simulink model "trafo1"  (Simulink 6.5)
settings: Solver=ode23t  StartTime=0.0  StopTime=1  RelTol=1e-3
undefined symbols (not defined in the file): powergui
libraries: powerlib x12, powerlib_extras x6
settings Model: Creator=RS  LastModifiedBy=RS

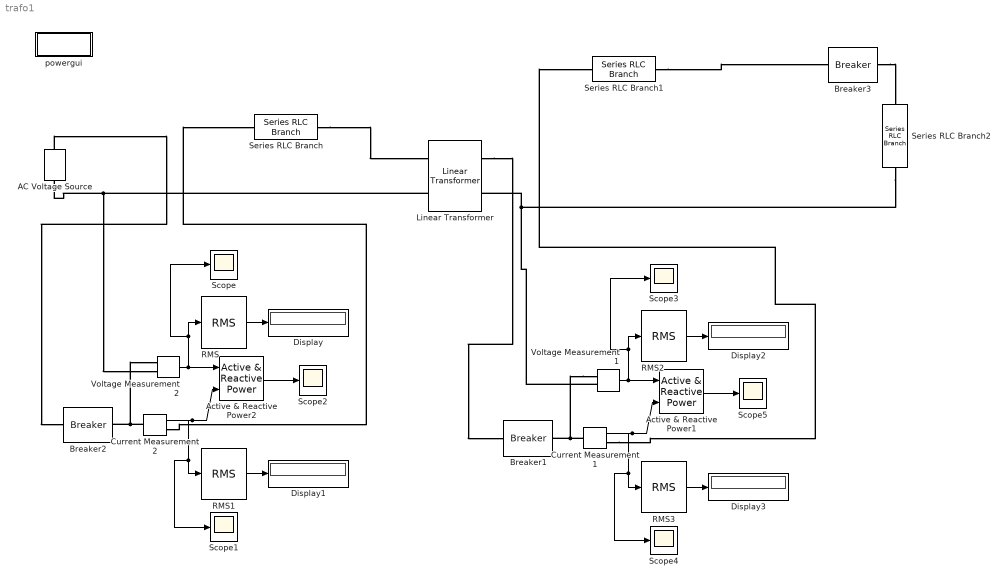
== system trafo1 ==
  AC Voltage Source : powerlib/Electrical Sources/AC Voltage Source  Orientation=up  DialogController=PMDialogs.PMDefaultMaskDlg  SystemSampleTime=-1  Amplitude=18172  Phase=0  Frequency=60  SampleTime=0  Measurements=None
  Active & Reactive Power1 : powerlib_extras/Measurements/Active & Reactive Power  DialogController=PMDialogs.PMDefaultMaskDlg  SystemSampleTime=-1  f1=60
  Active & Reactive Power2 : powerlib_extras/Measurements/Active & Reactive Power  DialogController=PMDialogs.PMDefaultMaskDlg  SystemSampleTime=-1  f1=60
  Breaker1 : powerlib/Elements/Breaker  DialogController=PMDialogs.PMDefaultMaskDlg  SystemSampleTime=-1  BreakerResistance=0.0001  InitialState=0  SnubberResistance=1e6  SnubberCapacitance=inf  SwitchingTimes="[ 0   2 ]"  External=off  Measurements=None  MoreParameters=off  NoBreakLoop=off
  Breaker2 : powerlib/Elements/Breaker  DialogController=PMDialogs.PMDefaultMaskDlg  SystemSampleTime=-1  BreakerResistance=0.0001  InitialState=0  SnubberResistance=1e6  SnubberCapacitance=inf  SwitchingTimes="[ 0   2 ]"  External=off  Measurements=None  MoreParameters=off  NoBreakLoop=off
  Breaker3 : powerlib/Elements/Breaker  DialogController=PMDialogs.PMDefaultMaskDlg  SystemSampleTime=-1  BreakerResistance=0.0001  InitialState=0  SnubberResistance=1e6  SnubberCapacitance=inf  SwitchingTimes="[ 0   2 ]"  External=off  Measurements=None  MoreParameters=off  NoBreakLoop=off
  Current Measurement1 : powerlib/Measurements/Current Measurement  DialogController=PMDialogs.PMDefaultMaskDlg  SystemSampleTime=-1  PhasorSimulation=off  OutputType=Complex  PSBequivalent=0
  Current Measurement2 : powerlib/Measurements/Current Measurement  DialogController=PMDialogs.PMDefaultMaskDlg  SystemSampleTime=-1  PhasorSimulation=off  OutputType=Complex  PSBequivalent=0
  Display{,1..3} (4 alike) : Display
  Linear Transformer : powerlib/Elements/Linear Transformer  DialogController=PMDialogs.PMDefaultMaskDlg  PhysicalDomain=powersysdomain  SubClassName=unknown  LeftPortType=p1  RightPortType=p1  LConnTagsString=a|b  RConnTagsString=A|B  UNITS=SI  NominalPower=[ 100000 60 ]  winding1="[12000    7.55      0.095875]"  winding2="[2400   0.302     0.003835]"  ThreeWindings=off  winding3=[3.15e+005 0.7938 0.084225]  RmLm="[99999999   99999999]"  Measurements=None  DataType=on
  RMS{,1..3} (4 alike) : powerlib_extras/Measurements/RMS  DialogController=PMDialogs.PMDefaultMaskDlg  SystemSampleTime=-1  f1=60
  Scope{,1..5} (6 alike) : Scope
      Scope settings: MaxDataPoints=10000000  SampleInput=on  SampleTime=10e-6
      Scope1 settings: MaxDataPoints=10000000  SampleInput=on  SampleTime=10e-6
      Scope2 settings: SaveName=ScopeData2  MaxDataPoints=10000000  SampleInput=on  SampleTime=10e-6
      Scope3 settings: SaveName=ScopeData3  MaxDataPoints=10000000  SampleInput=on  SampleTime=10e-6
      Scope4 settings: SaveName=ScopeData4  MaxDataPoints=10000000  SampleInput=on  SampleTime=10e-6
      Scope5 settings: SaveName=ScopeData5  MaxDataPoints=10000000  SampleInput=on  SampleTime=10e-6
  Series RLC Branch : powerlib/Elements/Series RLC Branch  DialogController=PMDialogs.PMDefaultMaskDlg  PhysicalDomain=powersysdomain  SubClassName=unknown  LeftPortType=p1  RightPortType=p1  LConnTagsString=__new0  RConnTagsString=__new0  BranchType=RL  Resistance=15.1  Inductance=0.17  SetiL0=off  InitialCurrent=0  Capacitance=1e-6  Setx0=off  InitialVoltage=0  Measurements=None
  Series RLC Branch1 : powerlib/Elements/Series RLC Branch  DialogController=PMDialogs.PMDefaultMaskDlg  PhysicalDomain=powersysdomain  SubClassName=unknown  LeftPortType=p1  RightPortType=p1  LConnTagsString=__new0  RConnTagsString=__new0  BranchType=RL  Resistance=1.27  Inductance=0.0047  SetiL0=off  InitialCurrent=0  Capacitance=1e-6  Setx0=off  InitialVoltage=0  Measurements=None
  Series RLC Branch2 : powerlib/Elements/Series RLC Branch  Orientation=down  DialogController=PMDialogs.PMDefaultMaskDlg  PhysicalDomain=powersysdomain  SubClassName=unknown  LeftPortType=p1  RightPortType=p1  LConnTagsString=__new0  RConnTagsString=__new0  BranchType=RL  Resistance=44.045  Inductance=0.0877  SetiL0=off  InitialCurrent=0  Capacitance=1e-6  Setx0=off  InitialVoltage=0  Measurements=None
  Voltage Measurement1 : powerlib/Measurements/Voltage Measurement  DialogController=PMDialogs.PMDefaultMaskDlg  SystemSampleTime=-1  PhasorSimulation=off  OutputType=Complex  PSBequivalent=0
  Voltage Measurement2 : powerlib/Measurements/Voltage Measurement  DialogController=PMDialogs.PMDefaultMaskDlg  SystemSampleTime=-1  PhasorSimulation=off  OutputType=Complex  PSBequivalent=0
  powergui : Subsystem  AncestorBlock=powerlib/powergui  InitFcn=powergui( 'InitFcn_Callback' , gcb , 0 , [ ] );  mask(PSB option menu block){SimulationMode=Continuous, SampleTime=50e-6, echomessages=off, RestoreLinks=warning, x0status=blocks, Frange=[0:2:500], Ylog=off, Xlog=on, ShowGrid=off, save=off, variable=ZData, structure=, ZoomFFT=on, StartTime=0.0, cycles=1, DisplayStyle=1, fundamental=60, FreqAxis=off, MaxFrequency=1000, frequencyindice=60, frequencyindicesteady=1, RmsSteady=1, display=off, Ts=0, frequency=60, methode=off, HookPort=off, Interpol=off}
      mask prompts: SimulationMode "Simulation mode"; SampleTime "Sample time Ts (when simulation mode is Discrete) (s)"; echomessages "Echo  Messages"; RestoreLinks "Restore disabled links"; x0status "Initial electrical states status"; Frange "Impedance tool: Frequency Range"; Ylog "Impedance tool: Log impedance"; Xlog "Impedance tool: log Frequency"; ShowGrid "Impedance tool: grid"; save "Impedance tool: Save Data To Workspace"; variable "Impedance tool: Variable Name"; structure "Structure Name (PSBFFTSCOPE)"; ZoomFFT "ZoomFFT (PSBFFTSCOPE)"; StartTime "Start Time (PSBFFTSCOPE)"; cycles "Cycles (PSBFFTSCOPE)"; DisplayStyle "Display style (PSBFFTSCOPE)"; fundamental "Fundamental (PSBFFTSCOPE)"; FreqAxis "Frequency Axis (PSBFFTSCOPE)"; MaxFrequency "Max Frequency (PSBFFTSCOPE)"; frequencyindice "Load flow frequency (Hz)"; frequencyindicesteady "Frequency indice (STEADYSTATE)"; RmsSteady "RMS display (STEADYSTATE)"; display "Display Results"; Ts "OBSOLETE 1"; frequency "Phasor frequency (Hz)"; methode "Phasor simulation"; HookPort "Hook port"; Interpol "Interpolate"
      mask init:
      | powerlibroot = which('powersysdomain');
      | PSBroot = powerlibroot(1:end-16);
      | %
      | switch SimulationMode
      | 	case 1
      | 		message=sprintf('Continuous');
      | 	case 2
      |         SampleTimeeval=evalin('base',SampleTime,'NaN');
      |         if isnan(SampleTimeeval)
      |             message=sprintf('Warning !!,\nUndefined sample time');
      |         else
      |             message=sprintf('Discrete,\nTs = %.4g s.',SampleTimeeval);
      |         end
      | 	case 3
      | 		message=sprintf('Phasors');
      | end
      | if strcmp(bdroot,'powerlib')
      |   message='powergui';
      | end
      | power_initmask();
      settings: CopyFcn=powergui( 'Copy_Callback' , gcb , 0 , [ ] );  ModelCloseFcn=powergui( 'CloseButton_Callback' , gcb , [ ] , [ ] );  PreSaveFcn=powergui( 'CloseButton_Callback' , gcb , [ ] , [ ] );  NameChangeFcn=powergui( 'NameChangeFcn_Callback' , gcb , 0 , [ ] );
      settings: DeleteFcn=|
      | powergui( 'Copy_Callback' , gcb , 1 , [ ] );
      | powergui( 'CloseButton_Callback' , gcb , [ ] , [ ] );
      settings: OpenFcn=|
      | if (power_openblockproxy ('secondary'))
      | powergui(gcb,'PM')
      | end;
      mask Help: web(psbhelp)
      mask StyleString: popup(Continuous|Discrete|Phasor),edit,checkbox,popup(yes|warning|no),popup(blocks|steady|zero),edit,checkbox,checkbox,checkbox,checkbox,edit,edit,checkbox,edit,edit,edit,edit,checkbox,edit,edit,edit,edit,checkbox,edit,edit,checkbox,checkbox,checkbox
      mask CallbackString: ||||||||||||||||||||||||||powergui('HookPort',[],[],gcb);|
      mask Display: disp(message)
  wires:
  Current Measurement2/1 -> Active & Reactive Power2/2, RMS1/1, Scope1/1
  Voltage Measurement2/1 -> Active & Reactive Power2/1, RMS/1, Scope/1
  Active & Reactive Power2/1 -> Scope2/1
  RMS/1 -> Display/1
  RMS1/1 -> Display1/1
  Current Measurement1/1 -> Active & Reactive Power1/2, RMS3/1, Scope4/1
  Voltage Measurement1/1 -> Active & Reactive Power1/1, RMS2/1, Scope3/1
  Active & Reactive Power1/1 -> Scope5/1
  RMS2/1 -> Display2/1
  RMS3/1 -> Display3/1
  connections:
  Current Measurement2/LConn1 -- Breaker2/RConn1 -- Voltage Measurement2/LConn1
  Voltage Measurement1/LConn1 -- Current Measurement1/LConn1 -- Breaker1/RConn1
  AC Voltage Source/RConn1 -- Breaker2/LConn1
  Linear Transformer/LConn2 -- AC Voltage Source/LConn1 -- Voltage Measurement2/LConn2
  Breaker3/RConn1 -- Series RLC Branch2/LConn1
  Voltage Measurement1/LConn2 -- Linear Transformer/RConn2 -- Series RLC Branch2/RConn1
  Linear Transformer/RConn1 -- Breaker1/LConn1
  Series RLC Branch1/RConn1 -- Breaker3/LConn1
  Series RLC Branch/RConn1 -- Linear Transformer/LConn1
  Current Measurement2/RConn1 -- Series RLC Branch/LConn1
  Current Measurement1/RConn1 -- Series RLC Branch1/LConn1

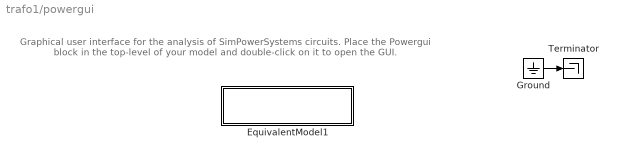
== system trafo1/powergui ==
  note: Graphical user interface for the analysis of  SimPowerSystems circuits.
      | Place the Powergui block in the top-level of your model and double-click
      | on it to open the GUI.
  EquivalentModel1 : Subsystem
      mask init:
      | SPS = get_param(gcbh,'UserData');
      | if isempty(SPS)
      |     A=0;
      |     B=0;
      |     C=0;
      |     D=0;
      |     x0=0;
      |     SwitchResistance=1;
      |     SwitchType=1;
      |     SwitchGateInitialValue=1;
      |     OutputsToResetToZero=1;
      | else
      | 	A=SPS.A;
      |     B=SPS.B;
      |     C=SPS.C;
      |     D=SPS.D;
      |     x0=SPS.x0;
      |     SwitchResistance=SPS.SwitchResistance;
      |     SwitchType=SPS.SwitchType;
      |     SwitchGateInitialValue=SPS.SwitchGateInitialValue;
      |     OutputsToResetToZero=SPS.YSwitchCurrent;
      | end
      mask Display:
      | color('blue')
      | disp('EQUIVALENT CIRCUIT')
  Ground : Ground
  Terminator : Terminator
  wires:
  Ground/1 -> Terminator/1

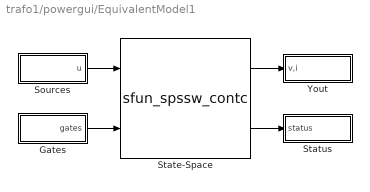
== system trafo1/powergui/EquivalentModel1 ==
  Gates : Subsystem
  Sources : Subsystem
  State-Space : S-Function  FunctionName=sfun_spssw_contc  Parameters=A, B, C, D, x0, SwitchResistance ,SwitchType, SwitchGateInitialValue, OutputsToResetToZero
  Status : Subsystem
  Yout : Subsystem
  wires:
  Gates/1(gates) -> State-Space/2
  Sources/1(u) -> State-Space/1
  State-Space/2 -> Status/1(status)
  State-Space/1 -> Yout/1(v,i)

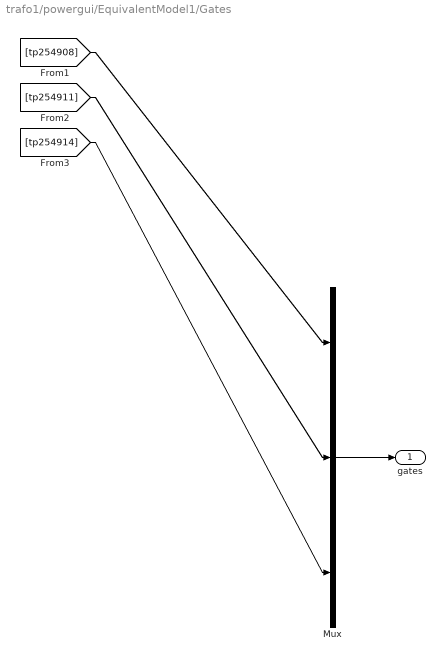
== system trafo1/powergui/EquivalentModel1/Gates ==
  Mux : Mux  Inputs=[1 1 1]
  gates : Outport
  wires:
  Mux/1 -> gates/1
  [tp254908] -> Mux/1
  [tp254911] -> Mux/2
  [tp254914] -> Mux/3

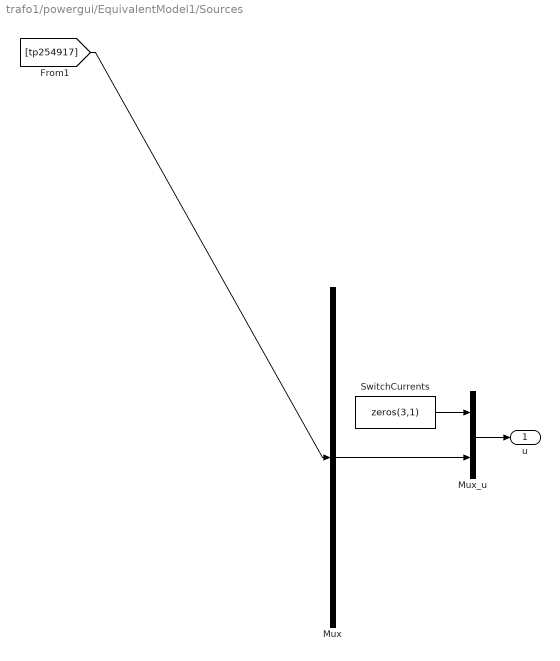
== system trafo1/powergui/EquivalentModel1/Sources ==
  Mux : Mux  Inputs=1
  Mux_u : Mux  Inputs=[3 1]
  SwitchCurrents : Constant  Value=zeros(3,1)  OutDataType=sfix(16)  ConRadixGroup=Use specified scaling  OutScaling=2^0  SampleTime=inf  FramePeriod=inf
  u : Outport
  wires:
  Mux/1 -> Mux_u/2
  SwitchCurrents/1 -> Mux_u/1
  Mux_u/1 -> u/1
  [tp254917] -> Mux/1

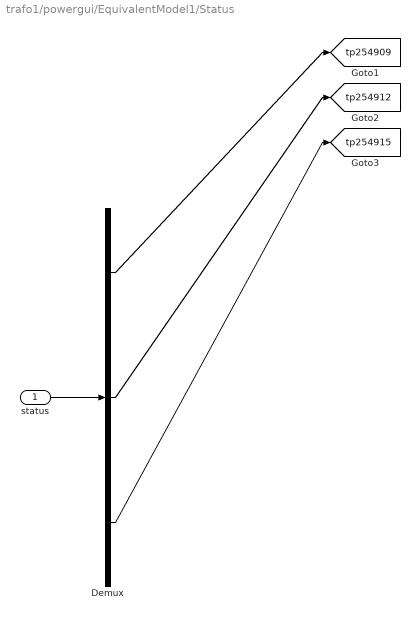
== system trafo1/powergui/EquivalentModel1/Status ==
  status : Inport
  Demux : Demux  Outputs=[1 1 1]
  tag scope: tp254909=global, tp254912=global, tp254915=global
  wires:
  status/1 -> Demux/1
  Demux/1 -> [tp254909]
  Demux/2 -> [tp254912]
  Demux/3 -> [tp254915]

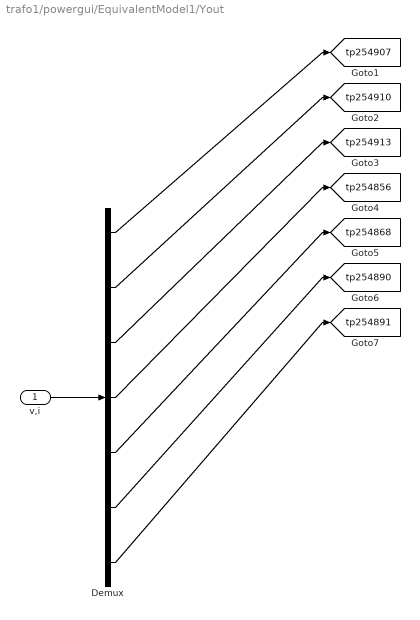
== system trafo1/powergui/EquivalentModel1/Yout ==
  v,i : Inport
  Demux : Demux  Outputs=[1 1 1 1 1 1 1]
  tag scope: tp254856=global, tp254868=global, tp254890=global, tp254891=global, tp254907=global, tp254910=global, tp254913=global
  wires:
  v,i/1 -> Demux/1
  Demux/1 -> [tp254907]
  Demux/2 -> [tp254910]
  Demux/3 -> [tp254913]
  Demux/4 -> [tp254856]
  Demux/5 -> [tp254868]
  Demux/6 -> [tp254890]
  Demux/7 -> [tp254891]
